simulink model "TRMS_Linear"  (Simulink 7.3)
settings: Solver=ode45  StartTime=0.0  StopTime=Exp.tsim  RelTol=1e-3
undefined symbols (not defined in the file): Exp, K, Obs, ss
libraries: simulink x1
settings Model: Creator=Greynosom  LastModifiedBy=sergarro
settings OptimizationCC: InitFltsAndDblsToZero=on
settings DebuggingCC: SaveWithParameterizedLinksMsg=none  SolverPrmCheckMsg=none
settings GRTTargetCC: TargetFcnLib=ansi_tfl_tmw.mat

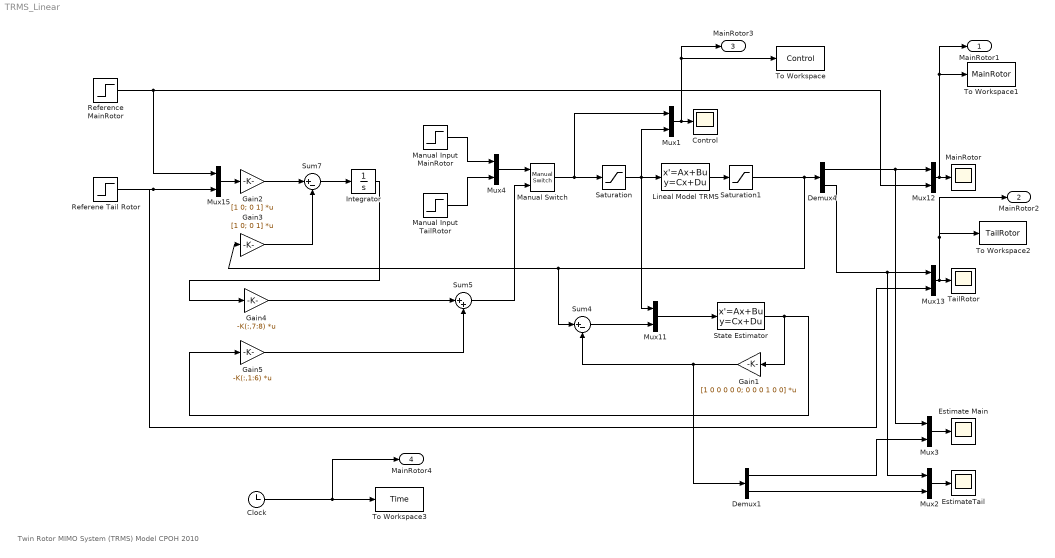
== system TRMS_Linear ==
  note: Twin Rotor MIMO System (TRMS) Model
      | CPOH 2010
  Clock : Clock
      settings: Decimation=10
  Control : Scope
      settings: SaveName=Control  DataFormat=Array  SampleInput=on  SampleTime=20/1000
  Demux1 : Demux  Outputs=2
  Demux4 : Demux  Outputs=2
  Estimate Main : Scope
      settings: TimeRange=20  YMin=-0.035  YMax=0.015  SaveName=ScopeData4
  EstimateTail : Scope
      settings: TimeRange=20  YMin=-0.035  YMax=0.015  SaveName=ScopeData3
  Gain1 : Gain  Gain=[1 0 0 0 0 0; 0 0 0 1 0 0]  Multiplication=Matrix(K*u) (u vector)  ParameterDataType=sfix(16)  ParameterScaling=2^0  OutDataType=sfix(16)  OutScaling=2^0
  Gain2 : Gain  Gain=[1 0; 0 1]  Multiplication=Matrix(K*u) (u vector)  ParameterDataType=sfix(16)  ParameterScaling=2^0  OutDataType=sfix(16)  OutScaling=2^0
  Gain3 : Gain  Gain=[1 0; 0 1]  Multiplication=Matrix(K*u) (u vector)  ParameterDataType=sfix(16)  ParameterScaling=2^0  OutDataType=sfix(16)  OutScaling=2^0
  Gain4 : Gain  Gain=-K(:,7:8)  Multiplication=Matrix(K*u) (u vector)  ParameterDataType=sfix(16)  ParameterScaling=2^0  OutDataType=sfix(16)  OutScaling=2^0
  Gain5 : Gain  Gain=-K(:,1:6)  Multiplication=Matrix(K*u) (u vector)  ParameterDataType=sfix(16)  ParameterScaling=2^0  OutDataType=sfix(16)  OutScaling=2^0
  Integrator : Integrator
  Lineal Model TRMS : StateSpace  A=ss.A  B=ss.B  C=ss.C  D=ss.D  X0=[0 0 0 0 0 0]
  MainRotor : Scope
      settings: YMin=-0.05  YMax=0.35  SaveName=MainRotor  DataFormat=Array  SampleInput=on  SampleTime=20/1000
  Manual Input MainRotor : Step  Time=0  After=0  SampleTime=0
  Manual Input TailRotor : Step  Time=0  After=0.1  SampleTime=0
  Manual Switch : simulink/Signal Routing/Manual Switch  SystemSampleTime=-1  sw=0  action=0  varsize=off
  Mux{1..4,11..13,15} (8 alike) : Mux  Inputs=2
  Reference MainRotor : Step  Time=Exp.MRstep  Before=Exp.MRini  After=Exp.MRfin  SampleTime=0
  Referene Tail Rotor : Step  Time=Exp.TRstep  Before=Exp.TRini  After=Exp.TRfin  SampleTime=0
  Saturation : Saturate  UpperLimit=1  LowerLimit=-1
  Saturation1 : Saturate  UpperLimit=pi  LowerLimit=-pi
  State Estimator : StateSpace  A=Obs.Ahat  B=Obs.Bhat  C=Obs.Chat  D=Obs.Dhat
  Sum4 : Sum  Inputs=|+-  OutDataType=sfix(16)  OutScaling=2^0
  Sum5 : Sum  Inputs=|++  OutDataType=sfix(16)  OutScaling=2^0
  Sum7 : Sum  Inputs=|+-  OutDataType=sfix(16)  OutScaling=2^0
  TailRotor : Scope
      settings: TimeRange=20  YMin=-0.035  YMax=0.015  SaveName=TailRotor  DataFormat=Array  SampleInput=on  SampleTime=20/1000
  To Workspace : ToWorkspace  VariableName=Control  SampleTime=20/1000  SaveFormat=Array
  To Workspace1 : ToWorkspace  VariableName=MainRotor  SampleTime=20/1000  SaveFormat=Array
  To Workspace2 : ToWorkspace  VariableName=TailRotor  SampleTime=20/1000  SaveFormat=Array
  To Workspace3 : ToWorkspace  VariableName=Time  SampleTime=20/1000  SaveFormat=Array
  MainRotor1 : Outport  OutDataType=fixdt(1, 16)  OutScaling=2^0
  MainRotor2 : Outport  Port=2  OutDataType=fixdt(1, 16)  OutScaling=2^0
  MainRotor3 : Outport  Port=3  OutDataType=fixdt(1, 16)  OutScaling=2^0
  MainRotor4 : Outport  Port=4  OutDataType=fixdt(1, 16)  OutScaling=2^0
  wires:
  State Estimator/1 -> Gain1/1, Gain5/1
  Mux11/1 -> State Estimator/1
  Sum4/1 -> Mux11/2
  Mux12/1 -> MainRotor/1, To Workspace1/1, MainRotor1/1
  Demux4/1 -> Mux12/1, Mux3/1
  Mux13/1 -> TailRotor/1, To Workspace2/1, MainRotor2/1
  Demux4/2 -> Mux13/1, Mux2/1
  Mux15/1 -> Gain2/1
  Reference MainRotor/1 -> Mux15/1, Mux12/2
  Referene Tail Rotor/1 -> Mux13/2, Mux15/2
  Gain2/1 -> Sum7/1
  Gain3/1 -> Sum7/2
  Sum7/1 -> Integrator/1
  Integrator/1 -> Gain4/1
  Gain4/1 -> Sum5/1
  Gain5/1 -> Sum5/2
  Saturation/1 -> Lineal Model TRMS/1, Mux1/2, Mux11/1
  Mux1/1 -> Control/1, To Workspace/1, MainRotor3/1
  Gain1/1 -> Sum4/2, Demux1/1
  Mux2/1 -> EstimateTail/1
  Mux3/1 -> Estimate Main/1
  Demux1/2 -> Mux2/2
  Demux1/1 -> Mux3/2
  Lineal Model TRMS/1 -> Saturation1/1
  Manual Switch/1 -> Saturation/1, Mux1/1
  Sum5/1 -> Manual Switch/2
  Mux4/1 -> Manual Switch/1
  Manual Input MainRotor/1 -> Mux4/1
  Manual Input TailRotor/1 -> Mux4/2
  Saturation1/1 -> Demux4/1, Gain3/1, Sum4/1
  Clock/1 -> To Workspace3/1, MainRotor4/1
